simulink model "pend"  (Simulink 6.6)
settings: Solver=ode45  StartTime=0.0  StopTime=10  MaxStep=0.05  RelTol=1e-3
undefined symbols (not defined in the file or in its folder): pend_control
settings Model: Creator=nsz  LastModifiedBy=nsz  ExtModeAutoUpdateStatusClock=off
settings SolverCC: InitialStep=0.01

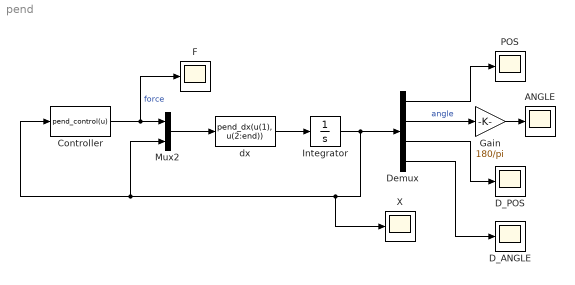
== system pend ==
  ANGLE : Scope
      settings: YMin=-17.5  YMax=30  SaveName=ScopeData2
  Controller : MATLABFcn  MATLABFcn=pend_control(u)  OutputDimensions=1
  D_ANGLE : Scope
      settings: YMin=-3.75  YMax=2  SaveName=ScopeData4
  D_POS : Scope
      settings: YMin=-3.75  YMax=2  SaveName=ScopeData3
  Demux : Demux
  F : Scope
      settings: YMin=-7.5  YMax=20  SaveName=ScopeData5
  Gain : Gain  Gain=180/pi
  Integrator : Integrator  InitialCondition=[0 0.5 0 0]
  Mux2 : Mux  Inputs=2
  POS : Scope
      settings: YMin=-3.75  YMax=2
  X : Scope
      settings: YMin=-3.75  YMax=2
  dx : MATLABFcn  MATLABFcn=pend_dx(u(1), u(2:end))  OutputDimensions=4
  wires:
  Mux2/1 -> dx/1
  Controller/1 -> Mux2/1, F/1  "force"
  Integrator/1 -> Controller/1, Mux2/2, X/1, Demux/1
  Demux/1 -> POS/1
  Demux/2 -> Gain/1  "angle"
  Demux/3 -> D_POS/1
  Demux/4 -> D_ANGLE/1
  dx/1 -> Integrator/1
  Gain/1 -> ANGLE/1
